simulink model "chap5_4sim"  (Simulink 6.3)
settings: Solver=ode45  StartTime=0.0  StopTime=20  RelTol=1e-3
values from neighbouring files (symbols this model uses):
  bp = 0.067    [chap5_5int.m]    (also in chap5_6int.m)
  Jp = 0.0030    (= 0.003)    [chap5_5int.m]    (also in chap5_6int.m)
  tol = 3    [chap5_12obv.m]    (also in chap5_13ctrl.m; chap5_13obv.m; chap5_5Q.m = 0.0004; chap5_5int.m = 0.001)
undefined symbols (not defined in the file or in its folder): den, num
libraries: simulink_extras x1
settings Model: Creator=a  LastModifiedBy=Administrator  ExtModeTrigMode=oneshot  ExtModeArmWhenConnect=off
settings DataIOCC: LimitDataPoints=off
settings OptimizationCC: BlockReduction=off  BooleanDataType=off
settings DebuggingCC: SolverPrmCheckMsg=none
settings HardwareCC: TargetUnknown=on

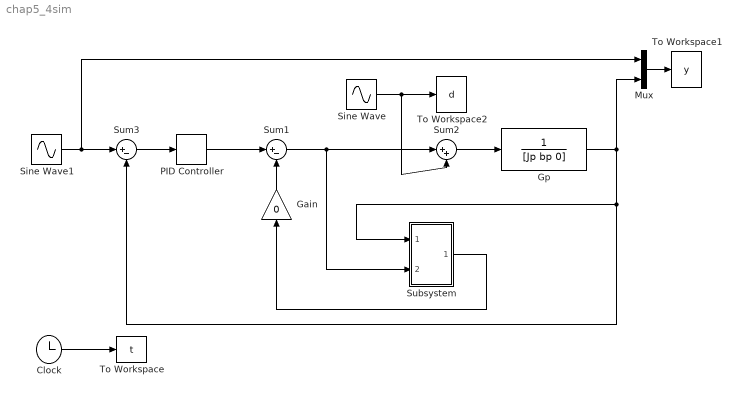
== system chap5_4sim ==
  Clock : Clock
      settings: Decimation=10
  Gain : Gain  Orientation=up  Gain=0
  Gp : TransferFcn  Denominator=[Jp bp 0]
  Mux : Mux  Inputs=2
  PID Controller : simulink_extras/Additional Linear/PID Controller  P=10  I=0  D=5
  Sine Wave : Sin  Amplitude=3  Frequency=2*pi  SampleTime=0
  Sine Wave1 : Sin  SampleTime=0
  Subsystem : Subsystem
  Sum1 : Sum  Inputs=|+-  SaturateOnIntegerOverflow=on  InputSameDT=on
  Sum2 : Sum  Inputs=|++  SaturateOnIntegerOverflow=on  InputSameDT=on
  Sum3 : Sum  Inputs=|+-  SaturateOnIntegerOverflow=on  InputSameDT=on
  To Workspace : ToWorkspace  VariableName=t  SampleTime=-1  SaveFormat=Array
  To Workspace1 : ToWorkspace  VariableName=y  SampleTime=-1  SaveFormat=Array
  To Workspace2 : ToWorkspace  VariableName=d  SampleTime=-1  SaveFormat=Array
  wires:
  PID Controller/1 -> Sum1/1
  Gp/1 -> Subsystem/1(In1), Sum3/2, Mux/2
  Sum2/1 -> Gp/1
  Sine Wave/1 -> Sum2/2, To Workspace2/1
  Sum1/1 -> Sum2/1, Subsystem/2(In2)
  Clock/1 -> To Workspace/1
  Subsystem/1(Out1) -> Gain/1
  Sum3/1 -> PID Controller/1
  Sine Wave1/1 -> Sum3/1, Mux/1
  Mux/1 -> To Workspace1/1
  Gain/1 -> Sum1/2

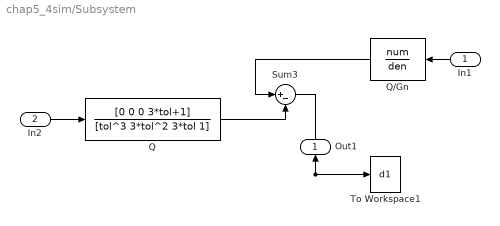
== system chap5_4sim/Subsystem ==
  In1 : Inport  Orientation=left
  In2 : Inport  Port=2
  Q : TransferFcn  Numerator=[0 0 0 3*tol+1]  Denominator=[tol^3 3*tol^2 3*tol 1]
  Q/Gn : TransferFcn  Orientation=left  Numerator=num  Denominator=den
  Sum3 : Sum  Inputs=|+-  SaturateOnIntegerOverflow=on  InputSameDT=on
  To Workspace1 : ToWorkspace  VariableName=d1  SampleTime=-1  SaveFormat=Array
  Out1 : Outport  Orientation=up
  wires:
  Q/Gn/1 -> Sum3/1
  Sum3/1 -> To Workspace1/1, Out1/1
  Q/1 -> Sum3/2
  In2/1 -> Q/1
  In1/1 -> Q/Gn/1
